simulink model "hil"  (R2024b)
settings: Solver=FixedStepAuto  StartTime=0.0  StopTime=10  FixedStep=0.001  RelTol=1e-3
undefined symbols (not defined in the file): CR
libraries: instrumentseriallib x3
settings Model: SimulationMode=accelerator  Creator=joedo  LastModifiedBy=joedo

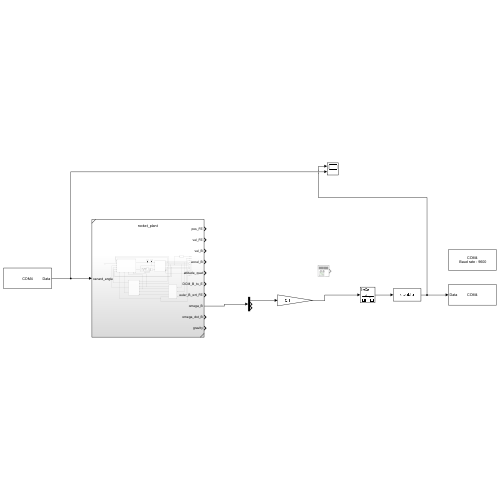
[thumbnail: Simulink's stored preview of the top-level diagram]
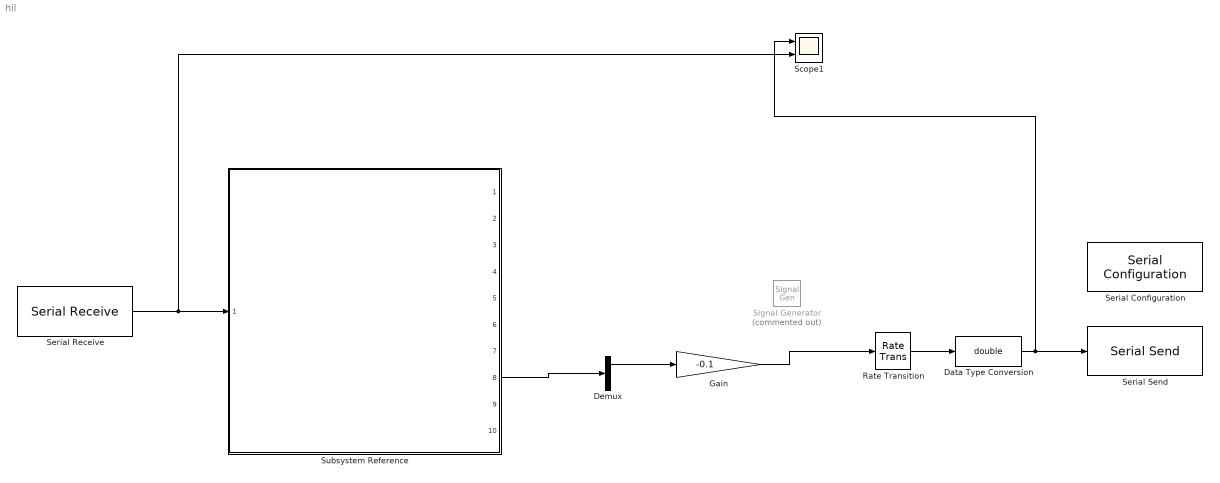
== system hil ==
  Data Type Conversion : DataTypeConversion  OutDataTypeStr=double  SaturateOnIntegerOverflow=off  RndMeth=Floor
  Demux : Demux  Outputs=3
  Gain : Gain  Gain=-0.1
  Rate Transition : RateTransition
  Scope1 : Scope  NumInputPorts=2
  Serial Configuration : instrumentseriallib/Serial Configuration  Priority=-200000  PortSel=COM4  Port=COM4  ComPort=COM4  BaudRate=9600  DataBits=8  Parity=none  StopBits=1  ByteOrder=little-endian  FlowControl=none  Timeout=10  SimulateUsing=Interpreted execution  BlockInModel=on  aMode=1
  Serial Receive : instrumentseriallib/Serial Receive  Priority=1  PortSel=COM4  Port=COM4  ComPort=COM4  DataType=double  SaveDataType=uint8  ToggleHeader=off  Header=[123]  ToggleDataSize=on  DataSize=[1]  ToggleTerminator=off  Terminator=CR ('\r')  CustomTerminator=[]  InputFormat=Column major  EnableBlockingMode=on  ActionDataUnavailable=Output last received value  ActionWhenDataUnavailable=Output last received value  CustomValue=0  SampleTime=0.001  SimulateUsing=Interpreted execution  BlockInModel=on  aMode=1
  Serial Send : instrumentseriallib/Serial Send  Priority=1  PortSel=COM4  Port=COM4  ComPort=COM4  Header=[]  Terminator=<none>  CustomTerminator=[]  EnableBlockingMode=on  SimulateUsing=Interpreted execution  BlockInModel=on  aMode=1
  Signal Generator : SignalGenerator  Commented=on  Frequency=2
  Subsystem Reference : Subsystem  ReferencedSubsystem=rocket_plant
  wires:
  Serial Receive/1 -> Scope1/2, Subsystem Reference/1
  Data Type Conversion/1 -> Scope1/1, Serial Send/1
  Rate Transition/1 -> Data Type Conversion/1
  Subsystem Reference/8 -> Demux/1
  Demux/1 -> Gain/1
  Gain/1 -> Rate Transition/1
